simulink model "dq0"  (R2023b)
settings: Solver=ode45  StartTime=0.0  StopTime=0.05  MaxStep=50e-6  RelTol=1e-3  EnableMultiTasking=on
PreLoadFcn:
  | Ts=50e-6;
InitFcn:
  | if ~exist('Ts','var')
  | Ts=50e-6;
  | end
libraries: spsThreePhaseProgrammableGeneratorLib x1, spsabctodq0Lib x1, simulink x1
settings Model: Creator=The MathWorks, Inc.  LastModifiedBy=marif
settings SolverCC: AlgebraicLoopSolver=TrustRegion
settings DataIOCC: LimitDataPoints=on  SaveFormat=Array  SaveOutput=off  SaveTime=off  ReturnWorkspaceOutputs=off
settings OptimizationCC: ExpressionDepthLimit=2147483647  LifeSpan=inf
settings DebuggingCC: UnderspecifiedInitializationDetection=Classic  MergeDetectMultiDrivingBlocksExec=none  FcnCallInpInsideContextMsg=warning  UnconnectedInputMsg=warning  UnconnectedOutputMsg=warning  UnconnectedLineMsg=warning  StateNameClashWarn=warning  SFUnexpectedBacktrackingDiag=warning  SFNoUnconditionalDefaultTransitionDiag=warning  SFExecutionAtInitializationDiag=none  ArithmeticOperatorsInVariantConditions=warning
settings HardwareCC: ProdBitPerPointer=32  ProdBitPerSizeT=32  ProdBitPerPtrDiffT=32  ProdLargestAtomicFloat=None  ProdIntDivRoundTo=Undefined  ProdEndianess=Unspecified  ProdWordSize=32  ProdHWDeviceType=32-bit Generic
settings ModelReferenceCC: EnableRefExpFcnMdlSchedulingChecks=on  PropagateSignalLabelsOutOfModel=off
settings SFSimCC: SimUseLocalCustomCode=off  CustomCodeUndefinedFunction=UseInterfaceOnly
settings RTWCC: RTWUseLocalCustomCode=off  DLArmComputeVersion=19.05
settings CodeAppCC: StateflowObjectComments=on
settings GRTTargetCC: TargetLangStandard=C89/C90 (ANSI)  CombineOutputUpdateFcns=off  GRTInterface=on
settings ConfigComp: CovMetricSettings=dw  CovSaveCumulativeToWorkspaceVar=on  CovSaveSingleToWorkspaceVar=on  CovExternalEMLEnable=off  CovSFcnEnable=off

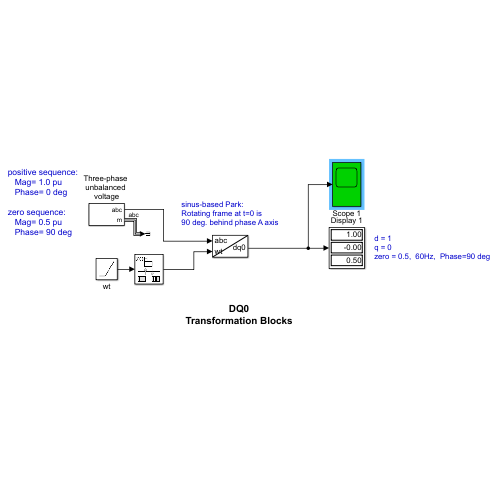
[thumbnail: Simulink's stored preview of the top-level diagram]
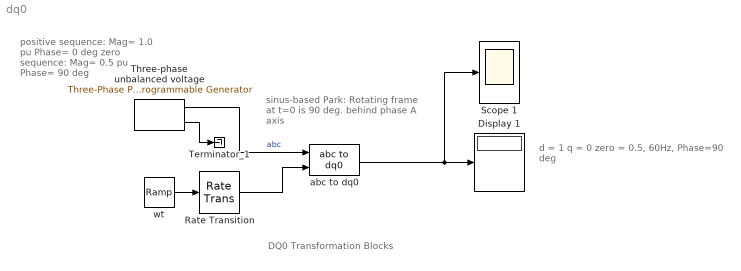
== system dq0 ==
  note: positive sequence:
      |    Mag= 1.0 pu
      |    Phase= 0 deg
      |
      | zero sequence:
      |    Mag= 0.5 pu
      |    Phase= 90 deg
  note: sinus-based Park:
      | Rotating frame at t=0 is
      | 90 deg. behind phase A axis
  note: DQ0
      |  Transformation Blocks
  note: d = 1
      | q = 0
      | zero = 0.5,  60Hz,  Phase=90 deg
  Display 1 : Display
      settings: Format=bank
  Rate Transition : RateTransition  OutPortSampleTime=Ts
  Scope 1 : Scope
  Terminator_1 : Terminator
  Three-phase unbalanced voltage : spsThreePhaseProgrammableGeneratorLib/Three-Phase Programmable Generator  Par_Vps="[1  0 60]"  VariationEntity=None  VariationType=Ramp  VariationStep=-0.5  VariationRate=10  VariationMag=0.3  VariationFreq=2  Par_Timing_Variation="[0.2  1.2]"  SinglePhase=on  Yampli=[1 0.2 1.2 1.0]  Xtime=[0 0.1 0.15 0.2]  HarmonicGeneration=on  Par_HarmoA="[1  0.5  90  0]"  Par_HarmoB="[1  0  0   2]"  Par_Timing_Harmo="[ 0  99]"  Ts=Ts
  abc to dq0 : spsabctodq0Lib/abc to dq0  Alignment=90 degrees behind phase A axis
  wt : simulink/Sources/Ramp  slope=2*pi*60  start=0  InitialOutput=0
  wires:
  wt/1 -> Rate Transition/1
  abc to dq0/1 -> Scope 1/1, Display 1/1
  Three-phase unbalanced voltage/1 -> abc to dq0/1  "abc"
  Three-phase unbalanced voltage/2 -> Terminator_1/1
  Rate Transition/1 -> abc to dq0/2
